simulink model "SDV_HIL"  (R2025a)
settings: Solver=VariableStepAuto  StartTime=0.0  StopTime=9999  FixedStep=0.001  RelTol=1e-3
undefined symbols (not defined in the file): Breakpoints_Fz, Cij, dspblkCoreblockFVToolHelper, eta, Fx_total_max, g, gcbh, Iz, lambda, lf, lr, mu, phi, R_eff, Tmax, xi
libraries: simulink_extras x30, slrealtimeiplib x17, slpidlib x16, simulink x10, SignalEditorBlockLib x6, dspstat3 x5, Solver_SF x3, sl3dlib x3
(part 1 of 5)
settings Model: SimulationMode=accelerator  Creator=zoan  LastModifiedBy=zoan

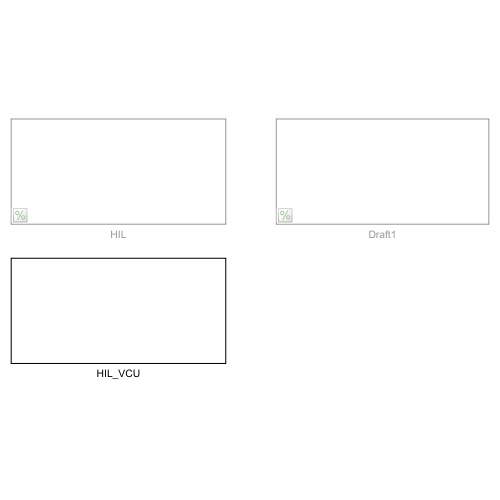
[thumbnail: Simulink's stored preview of the top-level diagram]
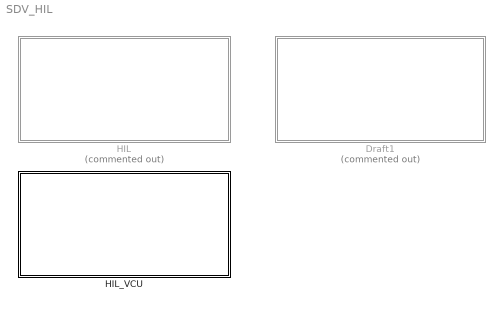
== system SDV_HIL ==
  Draft1 : Subsystem  Commented=on
  HIL : Subsystem  Commented=on
  HIL_VCU : Subsystem

== system SDV_HIL/Draft1 ==
  note: Communication (UDP Protocol)
  CarSim S-Function_video1 : Solver_SF/CarSim S-Function_video  Priority=1  SIMFILE=simfile.sim
      settings: SourceProductName=CarSim S-Function
  Communication System1 : Subsystem  Commented=on
  Connector1 : Subsystem
  Constant3 : Constant  Commented=on  Value=0
  Constant4 : Constant  Commented=on  Value=100
  Custom Trhottle2 : SignalEditorBlockLib/Signal Editor  Commented=on  FileName=Trottle.mat  ActiveScenario=Scenario  ActiveSignal=Signal 1  IsBus=off  OutputBusObjectStr=Bus: BusObject  SampleTime=0  ZeroCross=off  OutputAfterFinalValue=Setting to zero  Unit=inherit  PreserveSignalName=on  ApplySigPropsToAllScenarios=on  ApplySigPropsToAllSignals=off  SignalPropertySource=Dialog parameters
  Data Logger1 : Subsystem
  Driver Logi G1 : Subsystem
  Gain1 : Gain
  Goto2 : Goto  Commented=on  GotoTag=initialCondition  TagVisibility=global
  Sensor1 : Subsystem
  Speed - > Torque1 : Subsystem
  Steering Input1 : Subsystem
  Subsystem1 : Subsystem  Commented=on
  "UDP Receive ZCU -> PC1" : Subsystem
  "UDP Transmit PC -> VCU1" : Subsystem
  VCU Com1 : Subsystem  Commented=on
  tag scope: TqDrive=global
  wires:
  [Fz] -> "UDP Transmit PC -> VCU1"/7(Fz)
  [Vy] -> "UDP Transmit PC -> VCU1"/3(Vy)
  CarSim S-Function_video1/3 -> Sensor1/3(In3)
  [Vx] -> "UDP Transmit PC -> VCU1"/8(Spd)
  Connector1/1(Throttle) -> "UDP Transmit PC -> VCU1"/1(Throttle)
  Speed - > Torque1/1(TqDrive) -> CarSim S-Function_video1/1, [TqDrive]
  "UDP Receive ZCU -> PC1"/1(vxWheel_Ref) -> Speed - > Torque1/1(VxWheel_Ref)
  Steering Input1/1(Str) -> "UDP Transmit PC -> VCU1"/9(Str)
  Gain1/1 -> CarSim S-Function_video1/3
  [ThrottlePXN] -> Connector1/1(In1)
  [Vx] -> "UDP Transmit PC -> VCU1"/2(Vx)
  [yawrate] -> "UDP Transmit PC -> VCU1"/5(r)
  CarSim S-Function_video1/2 -> Sensor1/2(In2)
  Constant3/1 -> Goto2/1
  [Fy] -> "UDP Transmit PC -> VCU1"/6(Fy)
  [Brake_pedal] -> CarSim S-Function_video1/2
  CarSim S-Function_video1/1 -> Sensor1/1(In1)
  [AngWheel] -> "UDP Transmit PC -> VCU1"/4(AngWheel)
  "UDP Receive ZCU -> PC1"/2(AngWheel) -> Gain1/1

== system SDV_HIL/HIL ==
  note: Communication (UDP Protocol)
  CarSim S-Function_video : Solver_SF/CarSim S-Function_video  Priority=1  SIMFILE=simfile.sim
      settings: SourceProductName=CarSim S-Function
  Data Logger : Subsystem
  Driver : Subsystem
  Sensor : Subsystem
  "Speed -> Torque" : Subsystem
  "UDP Receive ZCU -> PC" : Subsystem
  "UDP Transmit PC -> VCU" : Subsystem
  wires:
  [BrakePXN] -> CarSim S-Function_video/2
  CarSim S-Function_video/1 -> Sensor/1(In1)
  "Speed -> Torque"/1(TqDrive) -> CarSim S-Function_video/1
  [Fz] -> "UDP Transmit PC -> VCU"/7(Fz)
  [Fy] -> "UDP Transmit PC -> VCU"/6(Fy)
  [AngWheel] -> "UDP Transmit PC -> VCU"/4(AngWheel)
  [Vx] -> "UDP Transmit PC -> VCU"/8(Spd)
  Driver/1(Throttle) -> "UDP Transmit PC -> VCU"/1(Throttle)
  [Vx] -> "UDP Transmit PC -> VCU"/2(Vx)
  [yawrate] -> "UDP Transmit PC -> VCU"/5(r)
  "UDP Receive ZCU -> PC"/2(AngWheel) -> CarSim S-Function_video/3
  CarSim S-Function_video/2 -> Sensor/2(In2)
  CarSim S-Function_video/3 -> Sensor/3(In3)
  [Vy] -> "UDP Transmit PC -> VCU"/3(Vy)
  "UDP Receive ZCU -> PC"/1(vxWheel_Ref) -> "Speed -> Torque"/1(VxWheel_Ref)
  Driver/2(Steer) -> "UDP Transmit PC -> VCU"/9(Str)

== system SDV_HIL/HIL_VCU ==
  note: Communication (UDP Protocol)
  CarSim S-Function_video : Solver_SF/CarSim S-Function_video  Priority=1  SIMFILE=simfile.sim
      settings: SourceProductName=CarSim S-Function
  Data Logger : Subsystem
  Sensor : Subsystem
  "Speed -> Torque" : Subsystem
  "UDP Receive ZCU -> PC" : Subsystem
  "UDP Receive Brake VCU -> PC" : Subsystem
  "UDP Transmit PC -> VCU" : Subsystem
  wires:
  CarSim S-Function_video/1 -> Sensor/1(In1)
  "Speed -> Torque"/1(TqDrive) -> CarSim S-Function_video/1
  "UDP Receive ZCU -> PC"/2(AngWheel) -> CarSim S-Function_video/3
  CarSim S-Function_video/2 -> Sensor/2(In2)
  CarSim S-Function_video/3 -> Sensor/3(In3)
  "UDP Receive ZCU -> PC"/1(vxWheel_Ref) -> "Speed -> Torque"/1(VxWheel_Ref)
  [Vx] -> "UDP Transmit PC -> VCU"/1(Vx)
  "UDP Receive Brake VCU -> PC"/1(Brake) -> CarSim S-Function_video/2
  [Vy] -> "UDP Transmit PC -> VCU"/2(Vy)
  [AngWheel] -> "UDP Transmit PC -> VCU"/3(AngWheel)
  [yawrate] -> "UDP Transmit PC -> VCU"/4(r)
  [Fz] -> "UDP Transmit PC -> VCU"/5(Fy)
  [Fy] -> "UDP Transmit PC -> VCU"/6(Fz)
  [VxWheel] -> "UDP Transmit PC -> VCU"/7(VxWheel)

== system SDV_HIL/Draft1/Communication System1 ==

== system SDV_HIL/Draft1/Connector1 ==
  In1 : Inport
  Throttle : Outport
  wires:
  In1/1 -> Throttle/1

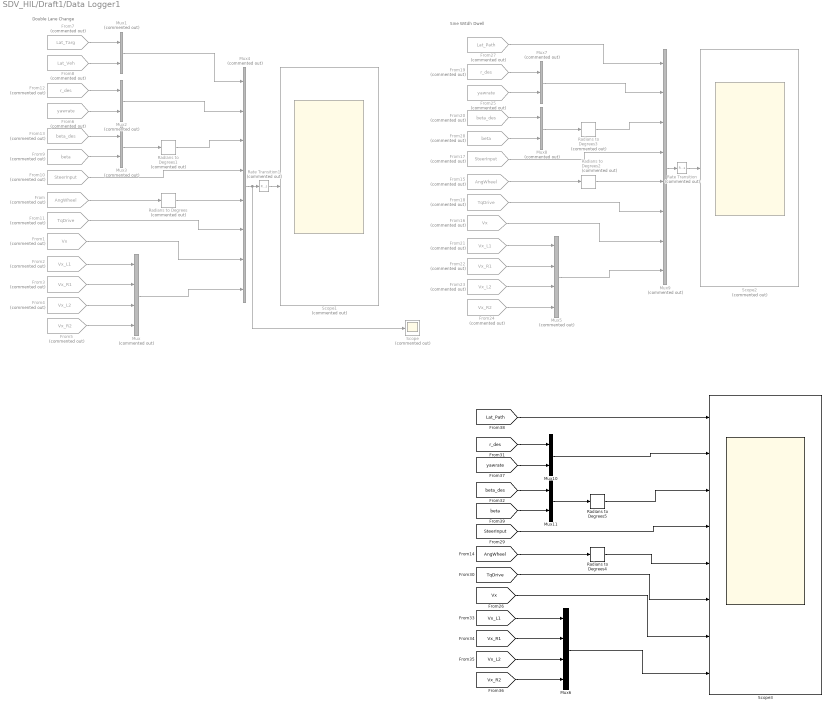
== system SDV_HIL/Draft1/Data Logger1 ==
  note: Sine Witdh Dwell
  note: Double Lane Change
  From : From  Commented=on  GotoTag=AngWheel  TagVisibility=global
  From1 : From  Commented=on  GotoTag=Vx  TagVisibility=global
  From10 : From  Commented=on  GotoTag=SteerInput  TagVisibility=global
  From11 : From  Commented=on  GotoTag=TqDrive  TagVisibility=global
  From12 : From  Commented=on  GotoTag=r_des  TagVisibility=global
  From13 : From  Commented=on  GotoTag=beta_des  TagVisibility=global
  From15 : From  Commented=on  GotoTag=AngWheel  TagVisibility=global
  From16 : From  Commented=on  GotoTag=Vx  TagVisibility=global
  From17 : From  Commented=on  GotoTag=SteerInput  TagVisibility=global
  From18 : From  Commented=on  GotoTag=TqDrive  TagVisibility=global
  From19 : From  Commented=on  GotoTag=r_des  TagVisibility=global
  From2 : From  Commented=on  GotoTag=Vx_L1  TagVisibility=global
  From20 : From  Commented=on  GotoTag=beta_des  TagVisibility=global
  From21 : From  Commented=on  GotoTag=Vx_L1  TagVisibility=global
  From22 : From  Commented=on  GotoTag=Vx_R1  TagVisibility=global
  From23 : From  Commented=on  GotoTag=Vx_L2  TagVisibility=global
  From24 : From  Commented=on  GotoTag=Vx_R2  TagVisibility=global
  From25 : From  Commented=on  GotoTag=yawrate  TagVisibility=global
  From27 : From  Commented=on  GotoTag=Lat_Path  TagVisibility=global
  From28 : From  Commented=on  GotoTag=beta  TagVisibility=global
  From3 : From  Commented=on  GotoTag=Vx_R1  TagVisibility=global
  From4 : From  Commented=on  GotoTag=Vx_L2  TagVisibility=global
  From5 : From  Commented=on  GotoTag=Vx_R2  TagVisibility=global
  From6 : From  Commented=on  GotoTag=yawrate  TagVisibility=global
  From7 : From  Commented=on  GotoTag=Lat_Targ  TagVisibility=global
  From8 : From  Commented=on  GotoTag=Lat_Veh  TagVisibility=global
  From9 : From  Commented=on  GotoTag=beta  TagVisibility=global
  Mux : Mux  Commented=on
  Mux{1..3,7..8} (5 alike) : Mux  Commented=on  Inputs=2
  Mux10 : Mux  Inputs=2
  Mux11 : Mux  Inputs=2
  Mux4 : Mux  Commented=on  Inputs=8
  Mux5 : Mux  Commented=on
  Mux6 : Mux
  Mux9 : Mux  Commented=on  Inputs=8
  Radians to Degrees{,1..3} (4 alike) : simulink_extras/Transformations/Radians to Degrees  Commented=on
  Radians to Degrees4 : simulink_extras/Transformations/Radians to Degrees
  Radians to Degrees5 : simulink_extras/Transformations/Radians to Degrees
  Rate Transition : RateTransition  Commented=on  OutPortSampleTime=0.0005
  Rate Transition1 : RateTransition  Commented=on  OutPortSampleTime=0.0005
  Scope : Scope  Commented=on
      settings: ActiveDisplayYMinimum=-386.40569302982072  ActiveDisplayYMaximum=478.46163200269257  DataLoggingVariableName=ScopeData6
  Scope1 : Scope  Commented=on
      settings: ActiveDisplayYMinimum=-502.14554579924982  ActiveDisplayYMaximum=1193.5717273110276  DataLoggingVariableName=DataPlot
  Scope2 : Scope  Commented=on
      settings: ActiveDisplayYMinimum=90.336925729103882  ActiveDisplayYMaximum=110.69965404556876  DataLoggingVariableName=DataPlot
  Scope3 : Scope  NumInputPorts=8
      settings: ActiveDisplayString=5  ActiveDisplayYMinimum=-20.053815552669828  ActiveDisplayYMaximum=12.34951779667281  YLabel=Wheel Steer angle (deg)  DataLoggingDecimation=10  DataLoggingVariableName=DataPlot1
  wires:
  From/1 -> Radians to Degrees/1
  From2/1 -> Mux/1
  From3/1 -> Mux/2
  From4/1 -> Mux/3
  From5/1 -> Mux/4
  From7/1 -> Mux1/1
  From8/1 -> Mux1/2
  From12/1 -> Mux2/1
  From6/1 -> Mux2/2
  From13/1 -> Mux3/1
  From9/1 -> Mux3/2
  Mux3/1 -> Radians to Degrees1/1
  Mux1/1 -> Mux4/1
  Mux2/1 -> Mux4/2
  Radians to Degrees1/1 -> Mux4/3
  From10/1 -> Mux4/4
  Radians to Degrees/1 -> Mux4/5
  From11/1 -> Mux4/6
  From1/1 -> Mux4/7
  Mux/1 -> Mux4/8
  Mux4/1 -> Scope/1, Rate Transition1/1
  Mux9/1 -> Rate Transition/1
  Mux5/1 -> Mux9/8
  From16/1 -> Mux9/7
  From18/1 -> Mux9/6
  Radians to Degrees2/1 -> Mux9/5
  From17/1 -> Mux9/4
  Radians to Degrees3/1 -> Mux9/3
  Mux7/1 -> Mux9/2
  From27/1 -> Mux9/1
  Mux8/1 -> Radians to Degrees3/1
  From28/1 -> Mux8/2
  From20/1 -> Mux8/1
  From25/1 -> Mux7/2
  From19/1 -> Mux7/1
  From24/1 -> Mux5/4
  From23/1 -> Mux5/3
  From22/1 -> Mux5/2
  From21/1 -> Mux5/1
  From15/1 -> Radians to Degrees2/1
  Rate Transition/1 -> Scope2/1
  Rate Transition1/1 -> Scope1/1
  [AngWheel] -> Radians to Degrees4/1
  [Vx_L1] -> Mux6/1
  [Vx_R1] -> Mux6/2
  [Vx_L2] -> Mux6/3
  [Vx_R2] -> Mux6/4
  [r_des] -> Mux10/1
  [yawrate] -> Mux10/2
  [beta_des] -> Mux11/1
  [beta] -> Mux11/2
  Mux11/1 -> Radians to Degrees5/1
  Radians to Degrees5/1 -> Scope3/3
  [Lat_Path] -> Scope3/1
  Mux10/1 -> Scope3/2
  [SteerInput] -> Scope3/4
  Radians to Degrees4/1 -> Scope3/5
  [TqDrive] -> Scope3/6
  [Vx] -> Scope3/7
  Mux6/1 -> Scope3/8

== system SDV_HIL/Draft1/Driver Logi G1 ==
  Add : Sum
  Add1 : Sum
  Constant : Constant  Value=50
  Constant1 : Constant  Value=6
  Demux : Demux
  Display : Display  Commented=on
  Display1 : Display  Commented=on
  Display{2,4..6} (4 alike) : Display
  Display3 : Display  Commented=on
  Gain3 : Gain  Gain=-6
  Gain4 : Gain  Gain=-50
  Gain5 : Gain  Gain=40
  MATLAB Function : MATLAB Function  TreatAsAtomicUnit=on
  Selector : Selector  InputPortWidth=25  IndexOptions=Index vector (dialog)  Indices=[1]  OutputSizes=1
  Simulation 3D Joystick : sl3dlib/Simulation 3D/Hardware Interface/Simulation 3D Joystick  joyid=1  adjustports=on  forcefeed=off
  Terminator : Terminator
  Terminator2 : Terminator
  tag scope: Brake_pedal=global, SteerPXN=global, ThrottlePXN=global
  wires:
  Simulation 3D Joystick/3 -> Terminator/1
  MATLAB Function/1(state) -> Display4/1
  Selector/1 -> MATLAB Function/1(btn)
  Gain5/1 -> [SteerPXN], Display2/1
  Add1/1 -> Display6/1, [Brake_pedal]
  Constant1/1 -> Add1/2
  Gain3/1 -> Add1/1
  Demux/3 -> Gain3/1
  Demux/2 -> Display3/1, Gain4/1
  Demux/1 -> Gain5/1
  Demux/4 -> Terminator2/1
  Simulation 3D Joystick/1 -> Demux/1, Display/1
  Gain4/1 -> Add/1
  Constant/1 -> Add/2
  Simulation 3D Joystick/2 -> Selector/1, Display1/1
  Add/1 -> Display5/1, [ThrottlePXN]

== system SDV_HIL/Draft1/Sensor1 ==
  In1 : Inport
  In2 : Inport  Port=2
  In3 : Inport  Port=3
  Display : Display  Commented=on
  Display1 : Display  Commented=on
  Display2 : Display  Commented=on
  Steering System : Subsystem
  Torque Vectoring : Subsystem
  Traction Control : Subsystem
  wires:
  In2/1 -> Steering System/1(In1), Display1/1
  In3/1 -> Traction Control/1(In1), Display2/1
  In1/1 -> Torque Vectoring/1(In1), Display/1

== system SDV_HIL/Draft1/Speed - > Torque1 ==
  VxWheel_Ref : Inport
  Demux : Demux
  Gain : Gain  Gain=4
  Mux : Mux
  PID Controller : slpidlib/PID Controller  Controller=PID  Form=Parallel  TimeDomain=Continuous-time  UseExternalTs=off  SampleTime=-1  IntegratorMethod=Forward Euler  FilterMethod=Forward Euler  ControllerParametersSource=internal  P=20  I=0.05  UseKiTs=off  D=1  UseExternalDerivativeSource=off  N=100  UseFilter=on  TunerSelectOption=Transfer Function Based (PID Tuner App)  InitialConditionSource=internal  InitialConditionForIntegrator=0  InitialConditionForFilter=0  DifferentiatorICPrevScaledInput=0  ExternalReset=none  TrackingMode=off  Kt=1  LimitOutput=off  SatLimitsSource=internal  UpperSaturationLimit=inf  LowerSaturationLimit=-inf  LinearizeAsGain=on  AntiWindupMode=none  Kb=1  LimitIntegrator=off  UpperIntegratorSaturationLimit=inf  LowerIntegratorSaturationLimit=-inf  POutMin=[]  POutMax=[]  IOutMin=[]  IOutMax=[]  DOutMin=[]  DOutMax=[]  NOutMin=[]  NOutMax=[]  SumOutMin=[]  SumOutMax=[]  SaturationOutMin=[]  SaturationOutMax=[]  PParamMin=[]  PParamMax=[]  IParamMin=[]  IParamMax=[]  DParamMin=[]  DParamMax=[]  NParamMin=[]  NParamMax=[]  KbParamMin=[]  KbParamMax=[]  KtParamMin=[]  KtParamMax=[]  KbOutMin=[]  KbOutMax=[]  KtOutMin=[]  KtOutMax=[]  IntegratorOutMin=[]  IntegratorOutMax=[]  FilterOutMin=[]  FilterOutMax=[]  SumI1OutMin=[]  SumI1OutMax=[]  SumI2OutMin=[]  SumI2OutMax=[]  SumI3OutMin=[]  SumI3OutMax=[]  SumI4OutMin=[]  SumI4OutMax=[]  SumDOutMin=[]  SumDOutMax=[]  DifferentiatorOutMin=[]  DifferentiatorOutMax=[]  FilterDiffOutCoefMin=[]  FilterDiffOutCoefMax=[]  ReciprocalOutMin=[]  ReciprocalOutMax=[]  SumDenOutMin=[]  SumDenOutMax=[]  SumNumOutMin=[]  SumNumOutMax=[]  DivideOutMin=[]  DivideOutMax=[]  UdiffTsProdOutMin=[]  UdiffTsProdOutMax=[]  NTsProdOutMin=[]  NTsProdOutMax=[]  UintegralTsProdOutMin=[]  UintegralTsProdOutMax=[]  UngainTsProdOutMin=[]  UngainTsProdOutMax=[]  ClampingZeroOutDataTypeStr=Inherit: Inherit via back propagation  ClampingZeroOutMin=[]  ClampingZeroOutMax=[]  FilterDenConstantOutDataTypeStr=Inherit: Inherit via back propagation  FilterDenConstantOutMin=[]  FilterDenConstantOutMax=[]  PCopyOutDataTypeStr=Inherit: Inherit via back propagation  PCopyOutMin=[]  PCopyOutMax=[]  NCopyOutDataTypeStr=Inherit: Inherit via back propagation  NCopyOutMin=[]  NCopyOutMax=[]  IntegratorContinuousStateAttributes=''  IntegratorStateMustResolveToSignalObject=off  IntegratorRTWStateStorageClass=Auto  FilterContinuousStateAttributes=''  FilterStateMustResolveToSignalObject=off  FilterRTWStateStorageClass=Auto  ParallelPVariant=InternalParameters  IdealPVariant=Disabled  IVariant=InternalParameters  DVariant=InternalParameters  IntegratorVariant=Continuous  SatVariant=Disabled  AWVariant=Passthrough  PCopyVariant=Disabled  TRVariant=Disabled  FdbkBlocksVariant=Forward  IdealPFdbkVariant=Disabled  SatFdbkVariant=Disabled  DerivativeFilterVariant=ContFilter  NVariant=InternalParameters  NCopyVariant=Disabled  FilterICVariant=InternalICsFilter  IntegratorICVariant=InternalICs  ExternalResetVariant=Disabled  TRSumVariant=Passthrough  SumFdbkVariant=Disabled  SumVariant=Sum_PID  TsampFilterVariant=InternalTs  TsampNgainVariant=Passthrough  TsampIntegralVariant=Disabled_SignalSpec  ExternalSaturationOutDataTypeStr=Inherit: Same as second input  DerivativeSourceVariant=ErrorSignal  PreIntVariant=InternalPreInt
  Saturation : Saturate  UpperLimit=256  LowerLimit=-256
  Scope : Scope  Commented=on  NumInputPorts=2
      settings: ActiveDisplayYMinimum=-100.56314203320845  ActiveDisplayYMaximum=848.44383025663615  DataLoggingVariableName=ScopeData8
  Scope1 : Scope  Commented=on  NumInputPorts=2
      settings: TimeSpan=10  ActiveDisplayYMinimum=-320  ActiveDisplayYMaximum=320  DataLoggingVariableName=ScopeData15
  Scope2 : Scope  Commented=on
      settings: ActiveDisplayYMinimum=-23.964257405589464  ActiveDisplayYMaximum=18.546534084894063  DataLoggingVariableName=ScopeData34
  Scope4 : Scope  Commented=on
      settings: ActiveDisplayYMinimum=-146.25  ActiveDisplayYMaximum=116.25  DataLoggingVariableName=ScopeData66
  Sum{,1..3} (4 alike) : Sum  Inputs=|+-
  TqDrive : Outport
  wires:
  [Vx_L1] -> Scope/2, Sum/2
  [Vx_R1] -> Sum1/2
  Sum1/1 -> Mux/2
  Sum2/1 -> Mux/3
  [Vx_L2] -> Sum2/2
  Sum3/1 -> Mux/4
  [Vx_R2] -> Sum3/2
  Sum/1 -> Mux/1
  Mux/1 -> Scope2/1, PID Controller/1
  PID Controller/1 -> Saturation/1
  Gain/1 -> Scope1/2, TqDrive/1
  Demux/2 -> Sum1/1
  Demux/3 -> Sum2/1
  Demux/4 -> Sum3/1
  Demux/1 -> Sum/1
  VxWheel_Ref/1 -> Scope4/1, Demux/1
  Saturation/1 -> Scope1/1, Gain/1

== system SDV_HIL/Draft1/Steering Input1 ==
  note: Skenario
  "DLC Lateral Target " : Subsystem  Commented=on
  DLC SteerDM : Subsystem  Commented=on
  Driver Logi G29 : Subsystem  Commented=on
  Gain : Gain  Gain=-1
  Manual Steering : Constant  Commented=on  Value=0
  Scope : Scope  Commented=on
      settings: ActiveDisplayYMinimum=-4.9999999999999991  ActiveDisplayYMaximum=45  DataLoggingVariableName=ScopeData2
  Signal Editor : SignalEditorBlockLib/Signal Editor  Commented=on  FileName=steerDM_DLC_vx100.mat  ActiveScenario=scenario  ActiveSignal=Steering  IsBus=off  OutputBusObjectStr=Bus: BusObject  SampleTime=0  ZeroCross=off  OutputAfterFinalValue=Setting to zero  Unit=inherit  PreserveSignalName=on  ApplySigPropsToAllScenarios=on  ApplySigPropsToAllSignals=off  SignalPropertySource=Dialog parameters
  Sine with Dwell : Subsystem  Commented=on
  Sine with Dwell shifted : Subsystem  Commented=on
  Slider : SliderBlock  ScaleMin=-40  ScaleMax=40
  Steering Custom : SignalEditorBlockLib/Signal Editor  Commented=on  FileName=SteeringTest.mat  ActiveScenario=Scenario  ActiveSignal=Signal 1  IsBus=off  OutputBusObjectStr=Bus: BusObject  SampleTime=0  ZeroCross=off  OutputAfterFinalValue=Setting to zero  Unit=inherit  PreserveSignalName=on  ApplySigPropsToAllScenarios=on  ApplySigPropsToAllSignals=off  SignalPropertySource=Dialog parameters
  Subsystem : Subsystem
  Str : Outport
  tag scope: SteerInput=global
  wires:
  Subsystem/1(Str) -> Str/1, Scope/1, [SteerInput]
  [SteerPXN] -> Gain/1
  Gain/1 -> Subsystem/1(In1)

== system SDV_HIL/Draft1/Subsystem1 ==
  note: Zone Control Unit
  Spd : Inport
  TqWheel : Inport  Port=2
  Mzd : Inport  Port=3
  Ang_reff : Inport  Port=4
  Braking1 : Constant  Value=0
  Motor1 : Subsystem
  Steering1 : Subsystem
      settings: PortSchema="{\"entries\":[{\"content\":{\"sides\":[{\"content\":{\"connectorIds\":[\"In1\"]},\"type\":\"ConnectorPlacement.EquallySpacedRectSide\",\"uuid\":\"adb0bf30-e73b-41b4-a208-76a28c974ff7\"},{\"content\":{\"connectorIds\":[\"Out1\"],\"side\":\"RIGHT\"},\"type\":\"ConnectorPlacement.EquallySpacedRectSide\",\"uuid\":\"cc4abc60-21d6-40e8-bf54-579eb1c50fc1\"},{\"content\":{\"connectorIds\":[\"In2\"],\"side\":\"TOP\"},\"type\":\"ConnectorPlacement.EquallySpacedRectSide\",\"uuid\":\"04732dee-d47d-454e-a8de-965e49d270ff\"}]},\"type\":\"ConnectorPlacement.EquallySpacedConnector\",\"uuid\":\"781362bb-60f7-4755-ab91-304bdf8ac197\"}],\"packageUris\":[\"http://schema.mathworks.com/mf0/Connector/R2020b\"],\"version\":\"1.0\"}"
  Torque to Speed Distribution1 : Subsystem
      settings: PortSchema="{\"entries\":[{\"content\":{\"sides\":[{\"content\":{\"connectorIds\":[\"In1\"]},\"type\":\"ConnectorPlacement.EquallySpacedRectSide\",\"uuid\":\"be15fe61-aaa9-4a20-91d9-47c89f8c78bb\"},{\"content\":{\"connectorIds\":[\"Out1\"],\"side\":\"RIGHT\"},\"type\":\"ConnectorPlacement.EquallySpacedRectSide\",\"uuid\":\"0d489c28-6df0-4c63-af6a-395fd75f26f4\"},{\"content\":{\"connectorIds\":[\"In2\"],\"side\":\"TOP\"},\"type\":\"ConnectorPlacement.EquallySpacedRectSide\",\"uuid\":\"15d17bd3-6c4e-4c2e-8205-0819f815bc2d\"}]},\"type\":\"ConnectorPlacement.EquallySpacedConnector\",\"uuid\":\"9692d941-d4e1-4d2b-a410-04ec1d2de3d9\"}],\"packageUris\":[\"http://schema.mathworks.com/mf0/Connector/R2020b\"],\"version\":\"1.0\"}"
  Out1 : Outport
  Out2 : Outport  Port=2
  Deg : Outport  Port=3
  tag scope: TqDrive=global
  wires:
  Spd/1 -> Torque to Speed Distribution1/2(Spd)
  Motor1/1(Out1) -> Out1/1, [TqDrive]
  Ang_reff/1 -> Steering1/1(Ang_reff)
  Torque to Speed Distribution1/1(SpdWheel) -> Motor1/1(SpdTCS)
  TqWheel/1 -> Torque to Speed Distribution1/1(TqWheel)
  Braking1/1 -> Out2/1
  Mzd/1 -> Steering1/2(Mzd)
  Steering1/1(Deg) -> Deg/1

== system SDV_HIL/Draft1/UDP Receive ZCU -> PC1 ==
  Display18 : Display
  Display26 : Display  Commented=on
  MATLAB Function : MATLAB Function  TreatAsAtomicUnit=on
  Median Filter : dspstat3/Median Filter  Commented=on  WindowLength=5  SimulateUsing=Interpreted execution
      settings: LibrarySourceBlock=|
      | dspfdesign/Median
      | Filter
  Mux : Mux
  Mux1 : Mux
  Rate Transition2 : RateTransition  OutPortSampleTime=0.0001
  Scope : Scope  Commented=on  NumInputPorts=2
      settings: TimeSpan=10  ActiveDisplayYMinimum=-148.76999999999998  ActiveDisplayYMaximum=138.92999999999998  DataLoggingVariableName=ScopeData62
  Scope1 : Scope  Commented=on
      settings: ActiveDisplayYMinimum=-50  ActiveDisplayYMaximum=-30  DataLoggingVariableName=ScopeData63
  Spd & Ang Convertion2 : Subsystem
  UDP Receive3 : slrealtimeiplib/UDP Receive  useHostTargetConn=off  ipAddress=10.252.62.212  localPort=4095  rcvWidth=7  rcvFmAny=on  fmAddress='10.252.62.51'  sampleTime=0.0001  enableMessage=off  maxPackets=1
  vxWheel_Ref : Outport
  AngWheel : Outport  Port=2
  wires:
  MATLAB Function/5(seqRecv) -> Display26/1
  UDP Receive3/2 -> Display18/1
  UDP Receive3/1 -> Rate Transition2/1
  Rate Transition2/1 -> MATLAB Function/1(payload)
  MATLAB Function/4(RR) -> Spd & Ang Convertion2/4(RR)
  MATLAB Function/3(RL) -> Spd & Ang Convertion2/3(RL)
  MATLAB Function/2(FR) -> Spd & Ang Convertion2/2(FR)
  MATLAB Function/1(FL) -> Spd & Ang Convertion2/1(FL)
  Spd & Ang Convertion2/1(ang_FL) -> Mux/1
  Spd & Ang Convertion2/2(ang_FR) -> Mux/2
  Spd & Ang Convertion2/3(ang_RL) -> Mux/3
  Spd & Ang Convertion2/4(ang_RR) -> Mux/4
  Mux/1 -> Scope1/1, AngWheel/1
  Mux1/1 -> Median Filter/1, Scope/1, vxWheel_Ref/1
  Spd & Ang Convertion2/5(vxWheel_FL) -> Mux1/1
  Spd & Ang Convertion2/6(vxWheel_FR) -> Mux1/2
  Spd & Ang Convertion2/7(vxWheel_RL) -> Mux1/3
  Spd & Ang Convertion2/8(vxWheel_RR) -> Mux1/4
  Median Filter/1 -> Scope/2

== system SDV_HIL/Draft1/UDP Transmit PC -> VCU1 ==
  note: UDP Send
      | Matlab -> ZCU
  Throttle : Inport
  Vx : Inport  Port=2
  Vy : Inport  Port=3
  AngWheel : Inport  Port=4
  r : Inport  Port=5
  Fy : Inport  Port=6
  Fz : Inport  Port=7
  Spd : Inport  Port=8
  Str : Inport  Port=9
  Data Type Conversion{,1..3} (4 alike) : DataTypeConversion  OutDataTypeStr=double  SaturateOnIntegerOverflow=off  RndMeth=Floor
  Display{,1,3,5} (4 alike) : Display
  Display4 : Display  Commented=on
  Rate Transition{1..4} (4 alike) : RateTransition  OutPortSampleTime=0.001
  Subsystem : Subsystem
  UDP Send1 : slrealtimeiplib/UDP Send  useHostTargetConn=off  toAddress='10.252.62.51'  toPort=5051  sampleTime=0.001  enableMessage=off  ipAddress=10.252.62.212  localPort=4095
  UDP Send2 : slrealtimeiplib/UDP Send  useHostTargetConn=off  toAddress='10.252.62.52'  toPort=5052  sampleTime=0.001  enableMessage=off  ipAddress=10.252.62.212  localPort=4095
  UDP Send3 : slrealtimeiplib/UDP Send  useHostTargetConn=off  toAddress='10.252.62.53'  toPort=5053  sampleTime=0.001  enableMessage=off  ipAddress=10.252.62.212  localPort=4095
  UDP Send4 : slrealtimeiplib/UDP Send  useHostTargetConn=off  toAddress='10.252.62.54'  toPort=5054  sampleTime=0.001  enableMessage=off  ipAddress=10.252.62.212  localPort=4095
  wires:
  Data Type Conversion2/1 -> UDP Send3/2, Display3/1
  Rate Transition3/1 -> UDP Send3/1
  Rate Transition4/1 -> UDP Send4/1
  Data Type Conversion3/1 -> UDP Send4/2, Display5/1
  Data Type Conversion1/1 -> Display1/1, UDP Send2/2
  Rate Transition2/1 -> UDP Send2/1
  Rate Transition1/1 -> UDP Send1/1
  Data Type Conversion/1 -> UDP Send1/2, Display/1
  Subsystem/1(payload1) -> Display4/1, Rate Transition1/1
  Throttle/1 -> Subsystem/1(Vx_des)
  Vx/1 -> Subsystem/2(Vx)
  Vy/1 -> Subsystem/3(Vy)
  AngWheel/1 -> Subsystem/4(AngWheel)
  r/1 -> Subsystem/5(r)
  Fy/1 -> Subsystem/6(Fy)
  Fz/1 -> Subsystem/7(Fz)
  Spd/1 -> Subsystem/8(Spd)
  Str/1 -> Subsystem/9(Str)
  Subsystem/2(len1) -> Data Type Conversion/1
  Subsystem/3(payload2) -> Rate Transition2/1
  Subsystem/4(len2) -> Data Type Conversion1/1
  Subsystem/5(payload3) -> Rate Transition3/1
  Subsystem/6(len3) -> Data Type Conversion2/1
  Subsystem/7(payload4) -> Rate Transition4/1
  Subsystem/8(len4) -> Data Type Conversion3/1

== system SDV_HIL/Draft1/VCU Com1 ==
  UDP Receive <- VCU1 : Subsystem
  "UDP Send -> VCU1" : Subsystem

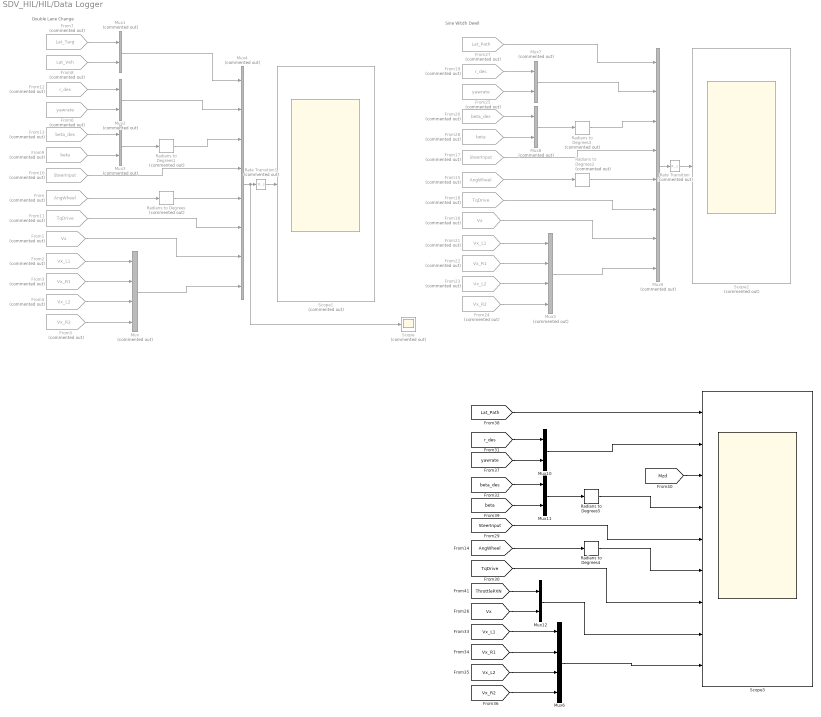
== system SDV_HIL/HIL/Data Logger ==
  note: Sine Witdh Dwell
  note: Double Lane Change
  From : From  Commented=on  GotoTag=AngWheel  TagVisibility=global
  From1 : From  Commented=on  GotoTag=Vx  TagVisibility=global
  From10 : From  Commented=on  GotoTag=SteerInput  TagVisibility=global
  From11 : From  Commented=on  GotoTag=TqDrive  TagVisibility=global
  From12 : From  Commented=on  GotoTag=r_des  TagVisibility=global
  From13 : From  Commented=on  GotoTag=beta_des  TagVisibility=global
  From15 : From  Commented=on  GotoTag=AngWheel  TagVisibility=global
  From16 : From  Commented=on  GotoTag=Vx  TagVisibility=global
  From17 : From  Commented=on  GotoTag=SteerInput  TagVisibility=global
  From18 : From  Commented=on  GotoTag=TqDrive  TagVisibility=global
  From19 : From  Commented=on  GotoTag=r_des  TagVisibility=global
  From2 : From  Commented=on  GotoTag=Vx_L1  TagVisibility=global
  From20 : From  Commented=on  GotoTag=beta_des  TagVisibility=global
  From21 : From  Commented=on  GotoTag=Vx_L1  TagVisibility=global
  From22 : From  Commented=on  GotoTag=Vx_R1  TagVisibility=global
  From23 : From  Commented=on  GotoTag=Vx_L2  TagVisibility=global
  From24 : From  Commented=on  GotoTag=Vx_R2  TagVisibility=global
  From25 : From  Commented=on  GotoTag=yawrate  TagVisibility=global
  From27 : From  Commented=on  GotoTag=Lat_Path  TagVisibility=global
  From28 : From  Commented=on  GotoTag=beta  TagVisibility=global
  From3 : From  Commented=on  GotoTag=Vx_R1  TagVisibility=global
  From4 : From  Commented=on  GotoTag=Vx_L2  TagVisibility=global
  From5 : From  Commented=on  GotoTag=Vx_R2  TagVisibility=global
  From6 : From  Commented=on  GotoTag=yawrate  TagVisibility=global
  From7 : From  Commented=on  GotoTag=Lat_Targ  TagVisibility=global
  From8 : From  Commented=on  GotoTag=Lat_Veh  TagVisibility=global
  From9 : From  Commented=on  GotoTag=beta  TagVisibility=global
  Mux : Mux  Commented=on
  Mux{1..3,7..8} (5 alike) : Mux  Commented=on  Inputs=2
  Mux10 : Mux  Inputs=2
  Mux11 : Mux  Inputs=2
  Mux12 : Mux  Inputs=2
  Mux4 : Mux  Commented=on  Inputs=8
  Mux5 : Mux  Commented=on
  Mux6 : Mux
  Mux9 : Mux  Commented=on  Inputs=8
  Radians to Degrees{,1..3} (4 alike) : simulink_extras/Transformations/Radians to Degrees  Commented=on
  Radians to Degrees4 : simulink_extras/Transformations/Radians to Degrees
  Radians to Degrees5 : simulink_extras/Transformations/Radians to Degrees
  Rate Transition : RateTransition  Commented=on  OutPortSampleTime=0.0005
  Rate Transition1 : RateTransition  Commented=on  OutPortSampleTime=0.0005
  Scope : Scope  Commented=on
      settings: ActiveDisplayYMinimum=-386.40569302982072  ActiveDisplayYMaximum=478.46163200269257  DataLoggingVariableName=ScopeData6
  Scope1 : Scope  Commented=on
      settings: ActiveDisplayYMinimum=-502.14554579924982  ActiveDisplayYMaximum=1193.5717273110276  DataLoggingVariableName=DataPlot
  Scope2 : Scope  Commented=on
      settings: ActiveDisplayYMinimum=90.336925729103882  ActiveDisplayYMaximum=110.69965404556876  DataLoggingVariableName=DataPlot
  Scope3 : Scope  NumInputPorts=9
      settings: TimeSpan=10  ActiveDisplayString=3  ActiveDisplayYMinimum=-593509.73040498013  ActiveDisplayYMaximum=954008.31003345363  YLabel=Mzd (Nm)  DataLoggingDecimation=10  DataLoggingVariableName=DataPlot1
  wires:
  From/1 -> Radians to Degrees/1
  From2/1 -> Mux/1
  From3/1 -> Mux/2
  From4/1 -> Mux/3
  From5/1 -> Mux/4
  From7/1 -> Mux1/1
  From8/1 -> Mux1/2
  From12/1 -> Mux2/1
  From6/1 -> Mux2/2
  From13/1 -> Mux3/1
  From9/1 -> Mux3/2
  Mux3/1 -> Radians to Degrees1/1
  Mux1/1 -> Mux4/1
  Mux2/1 -> Mux4/2
  Radians to Degrees1/1 -> Mux4/3
  From10/1 -> Mux4/4
  Radians to Degrees/1 -> Mux4/5
  From11/1 -> Mux4/6
  From1/1 -> Mux4/7
  Mux/1 -> Mux4/8
  Mux4/1 -> Scope/1, Rate Transition1/1
  Mux9/1 -> Rate Transition/1
  Mux5/1 -> Mux9/8
  From16/1 -> Mux9/7
  From18/1 -> Mux9/6
  Radians to Degrees2/1 -> Mux9/5
  From17/1 -> Mux9/4
  Radians to Degrees3/1 -> Mux9/3
  Mux7/1 -> Mux9/2
  From27/1 -> Mux9/1
  Mux8/1 -> Radians to Degrees3/1
  From28/1 -> Mux8/2
  From20/1 -> Mux8/1
  From25/1 -> Mux7/2
  From19/1 -> Mux7/1
  From24/1 -> Mux5/4
  From23/1 -> Mux5/3
  From22/1 -> Mux5/2
  From21/1 -> Mux5/1
  From15/1 -> Radians to Degrees2/1
  Rate Transition/1 -> Scope2/1
  Rate Transition1/1 -> Scope1/1
  [AngWheel] -> Radians to Degrees4/1
  [Vx_L1] -> Mux6/1
  [Vx_R1] -> Mux6/2
  [Vx_L2] -> Mux6/3
  [Vx_R2] -> Mux6/4
  [r_des] -> Mux10/1
  [yawrate] -> Mux10/2
  [beta_des] -> Mux11/1
  [beta] -> Mux11/2
  Mux11/1 -> Radians to Degrees5/1
  [Lat_Path] -> Scope3/1
  Mux10/1 -> Scope3/2
  Radians to Degrees5/1 -> Scope3/4
  [SteerInput] -> Scope3/5
  Radians to Degrees4/1 -> Scope3/6
  [TqDrive] -> Scope3/7
  Mux6/1 -> Scope3/9
  [Mzd] -> Scope3/3
  [ThrottlePXN] -> Mux12/1
  [Vx] -> Mux12/2
  Mux12/1 -> Scope3/8

== system SDV_HIL/HIL/Driver ==
  note: Skenario
  DLC SteerDM : Subsystem  Commented=on
  Gain : Gain  Gain=-1
  Logitech G29 : Subsystem
  Scope : Scope  Commented=on
      settings: ActiveDisplayYMinimum=-4.9999999999999991  ActiveDisplayYMaximum=45  DataLoggingVariableName=ScopeData2
  Sine with Dwell : Subsystem  Commented=on
  Subsystem : Subsystem
  Throttle : Outport
  Steer : Outport  Port=2
  tag scope: SteerInput=global
  wires:
  Gain/1 -> Subsystem/1(In1)
  [ThrottlePXN] -> Throttle/1
  Subsystem/1(Str) -> [SteerInput], Scope/1, Steer/1
  [SteerPXN] -> Gain/1

== system SDV_HIL/HIL/Sensor ==
  In1 : Inport
  In2 : Inport  Port=2
  In3 : Inport  Port=3
  Display : Display  Commented=on
  Display1 : Display  Commented=on
  Display2 : Display  Commented=on
  Steering System : Subsystem
  Torque Vectoring : Subsystem
  Traction Control : Subsystem
  wires:
  In2/1 -> Steering System/1(In1), Display1/1
  In3/1 -> Traction Control/1(In1), Display2/1
  In1/1 -> Torque Vectoring/1(In1), Display/1

== system SDV_HIL/HIL/Speed -> Torque ==
  VxWheel_Ref : Inport
  Demux : Demux
  Gain : Gain  Gain=4
  Mux : Mux
  PID Controller : slpidlib/PID Controller  Controller=PID  Form=Parallel  TimeDomain=Continuous-time  UseExternalTs=off  SampleTime=-1  IntegratorMethod=Forward Euler  FilterMethod=Forward Euler  ControllerParametersSource=internal  P=20  I=0.05  UseKiTs=off  D=1  UseExternalDerivativeSource=off  N=100  UseFilter=on  TunerSelectOption=Transfer Function Based (PID Tuner App)  InitialConditionSource=internal  InitialConditionForIntegrator=0  InitialConditionForFilter=0  DifferentiatorICPrevScaledInput=0  ExternalReset=none  TrackingMode=off  Kt=1  LimitOutput=off  SatLimitsSource=internal  UpperSaturationLimit=inf  LowerSaturationLimit=-inf  LinearizeAsGain=on  AntiWindupMode=none  Kb=1  LimitIntegrator=off  UpperIntegratorSaturationLimit=inf  LowerIntegratorSaturationLimit=-inf  POutMin=[]  POutMax=[]  IOutMin=[]  IOutMax=[]  DOutMin=[]  DOutMax=[]  NOutMin=[]  NOutMax=[]  SumOutMin=[]  SumOutMax=[]  SaturationOutMin=[]  SaturationOutMax=[]  PParamMin=[]  PParamMax=[]  IParamMin=[]  IParamMax=[]  DParamMin=[]  DParamMax=[]  NParamMin=[]  NParamMax=[]  KbParamMin=[]  KbParamMax=[]  KtParamMin=[]  KtParamMax=[]  KbOutMin=[]  KbOutMax=[]  KtOutMin=[]  KtOutMax=[]  IntegratorOutMin=[]  IntegratorOutMax=[]  FilterOutMin=[]  FilterOutMax=[]  SumI1OutMin=[]  SumI1OutMax=[]  SumI2OutMin=[]  SumI2OutMax=[]  SumI3OutMin=[]  SumI3OutMax=[]  SumI4OutMin=[]  SumI4OutMax=[]  SumDOutMin=[]  SumDOutMax=[]  DifferentiatorOutMin=[]  DifferentiatorOutMax=[]  FilterDiffOutCoefMin=[]  FilterDiffOutCoefMax=[]  ReciprocalOutMin=[]  ReciprocalOutMax=[]  SumDenOutMin=[]  SumDenOutMax=[]  SumNumOutMin=[]  SumNumOutMax=[]  DivideOutMin=[]  DivideOutMax=[]  UdiffTsProdOutMin=[]  UdiffTsProdOutMax=[]  NTsProdOutMin=[]  NTsProdOutMax=[]  UintegralTsProdOutMin=[]  UintegralTsProdOutMax=[]  UngainTsProdOutMin=[]  UngainTsProdOutMax=[]  ClampingZeroOutDataTypeStr=Inherit: Inherit via back propagation  ClampingZeroOutMin=[]  ClampingZeroOutMax=[]  FilterDenConstantOutDataTypeStr=Inherit: Inherit via back propagation  FilterDenConstantOutMin=[]  FilterDenConstantOutMax=[]  PCopyOutDataTypeStr=Inherit: Inherit via back propagation  PCopyOutMin=[]  PCopyOutMax=[]  NCopyOutDataTypeStr=Inherit: Inherit via back propagation  NCopyOutMin=[]  NCopyOutMax=[]  IntegratorContinuousStateAttributes=''  IntegratorStateMustResolveToSignalObject=off  IntegratorRTWStateStorageClass=Auto  FilterContinuousStateAttributes=''  FilterStateMustResolveToSignalObject=off  FilterRTWStateStorageClass=Auto  ParallelPVariant=InternalParameters  IdealPVariant=Disabled  IVariant=InternalParameters  DVariant=InternalParameters  IntegratorVariant=Continuous  SatVariant=Disabled  AWVariant=Passthrough  PCopyVariant=Disabled  TRVariant=Disabled  FdbkBlocksVariant=Forward  IdealPFdbkVariant=Disabled  SatFdbkVariant=Disabled  DerivativeFilterVariant=ContFilter  NVariant=InternalParameters  NCopyVariant=Disabled  FilterICVariant=InternalICsFilter  IntegratorICVariant=InternalICs  ExternalResetVariant=Disabled  TRSumVariant=Passthrough  SumFdbkVariant=Disabled  SumVariant=Sum_PID  TsampFilterVariant=InternalTs  TsampNgainVariant=Passthrough  TsampIntegralVariant=Disabled_SignalSpec  ExternalSaturationOutDataTypeStr=Inherit: Same as second input  DerivativeSourceVariant=ErrorSignal  PreIntVariant=InternalPreInt
  Saturation : Saturate  UpperLimit=256  LowerLimit=-100
  Scope : Scope  Commented=on  NumInputPorts=2
      settings: ActiveDisplayYMinimum=-100.56314203320845  ActiveDisplayYMaximum=848.44383025663615  DataLoggingVariableName=ScopeData8
  Scope1 : Scope  Commented=on  NumInputPorts=2
      settings: TimeSpan=10  ActiveDisplayYMinimum=-320  ActiveDisplayYMaximum=320  DataLoggingVariableName=ScopeData15
  Scope2 : Scope  Commented=on
      settings: ActiveDisplayYMinimum=-23.964257405589464  ActiveDisplayYMaximum=18.546534084894063  DataLoggingVariableName=ScopeData34
  Scope4 : Scope  Commented=on
      settings: ActiveDisplayYMinimum=-146.25  ActiveDisplayYMaximum=116.25  DataLoggingVariableName=ScopeData66
  Sum{,1..3} (4 alike) : Sum  Inputs=|+-
  TqDrive : Outport
  tag scope: TqDrive=global
  wires:
  [Vx_L1] -> Scope/2, Sum/2
  [Vx_R1] -> Sum1/2
  Sum1/1 -> Mux/2
  Sum2/1 -> Mux/3
  [Vx_L2] -> Sum2/2
  Sum3/1 -> Mux/4
  [Vx_R2] -> Sum3/2
  Sum/1 -> Mux/1
  Mux/1 -> Scope2/1, PID Controller/1
  PID Controller/1 -> Saturation/1
  Gain/1 -> [TqDrive], Scope1/2, TqDrive/1
  Demux/2 -> Sum1/1
  Demux/3 -> Sum2/1
  Demux/4 -> Sum3/1
  Demux/1 -> Sum/1
  VxWheel_Ref/1 -> Scope4/1, Demux/1
  Saturation/1 -> Scope1/1, Gain/1

== system SDV_HIL/HIL/UDP Receive ZCU -> PC ==
  Display18 : Display
  Display26 : Display  Commented=on
  Gain1 : Gain  Gain=-1
  MATLAB Function : MATLAB Function  TreatAsAtomicUnit=on
  Median Filter : dspstat3/Median Filter  Commented=on  WindowLength=5  SimulateUsing=Interpreted execution
      settings: LibrarySourceBlock=|
      | dspfdesign/Median
      | Filter
  Mux : Mux
  Mux1 : Mux
  Rate Transition2 : RateTransition  OutPortSampleTime=0.0001
  Scope : Scope  Commented=on  NumInputPorts=2
      settings: TimeSpan=10  ActiveDisplayYMinimum=-148.76999999999998  ActiveDisplayYMaximum=138.92999999999998  DataLoggingVariableName=ScopeData62
  Scope1 : Scope  Commented=on
      settings: ActiveDisplayYMinimum=-50  ActiveDisplayYMaximum=-30  DataLoggingVariableName=ScopeData63
  Spd & Ang Convertion2 : Subsystem
  UDP Receive3 : slrealtimeiplib/UDP Receive  useHostTargetConn=off  ipAddress=10.252.62.212  localPort=4095  rcvWidth=7  rcvFmAny=on  fmAddress='10.252.62.51'  sampleTime=0.0001  enableMessage=off  maxPackets=1
  vxWheel_Ref : Outport
  AngWheel : Outport  Port=2
  wires:
  MATLAB Function/5(seqRecv) -> Display26/1
  UDP Receive3/2 -> Display18/1
  UDP Receive3/1 -> Rate Transition2/1
  Rate Transition2/1 -> MATLAB Function/1(payload)
  MATLAB Function/4(RR) -> Spd & Ang Convertion2/4(RR)
  MATLAB Function/3(RL) -> Spd & Ang Convertion2/3(RL)
  MATLAB Function/2(FR) -> Spd & Ang Convertion2/2(FR)
  MATLAB Function/1(FL) -> Spd & Ang Convertion2/1(FL)
  Spd & Ang Convertion2/1(ang_FL) -> Mux/1
  Spd & Ang Convertion2/2(ang_FR) -> Mux/2
  Spd & Ang Convertion2/3(ang_RL) -> Mux/3
  Spd & Ang Convertion2/4(ang_RR) -> Mux/4
  Mux/1 -> Gain1/1
  Spd & Ang Convertion2/5(vxWheel_FL) -> Mux1/1
  Spd & Ang Convertion2/6(vxWheel_FR) -> Mux1/2
  Spd & Ang Convertion2/7(vxWheel_RL) -> Mux1/3
  Spd & Ang Convertion2/8(vxWheel_RR) -> Mux1/4
  Median Filter/1 -> Scope/2
  Mux1/1 -> Median Filter/1, vxWheel_Ref/1, Scope/1
  Gain1/1 -> Scope1/1, AngWheel/1

== system SDV_HIL/HIL/UDP Transmit PC -> VCU ==
  note: UDP Send
      | Matlab -> ZCU
  Throttle : Inport
  Vx : Inport  Port=2
  Vy : Inport  Port=3
  AngWheel : Inport  Port=4
  r : Inport  Port=5
  Fy : Inport  Port=6
  Fz : Inport  Port=7
  Spd : Inport  Port=8
  Str : Inport  Port=9
  Data Type Conversion{,1..3} (4 alike) : DataTypeConversion  OutDataTypeStr=double  SaturateOnIntegerOverflow=off  RndMeth=Floor
  Display{,1,3,5} (4 alike) : Display
  Display4 : Display  Commented=on
  Gain1 : Gain  Gain=-1
  Rate Transition{1..4} (4 alike) : RateTransition  OutPortSampleTime=0.001
  Subsystem : Subsystem
  UDP Send1 : slrealtimeiplib/UDP Send  useHostTargetConn=off  toAddress='10.252.62.51'  toPort=5051  sampleTime=0.001  enableMessage=off  ipAddress=10.252.62.212  localPort=4095
  UDP Send2 : slrealtimeiplib/UDP Send  useHostTargetConn=off  toAddress='10.252.62.52'  toPort=5052  sampleTime=0.001  enableMessage=off  ipAddress=10.252.62.212  localPort=4095
  UDP Send3 : slrealtimeiplib/UDP Send  useHostTargetConn=off  toAddress='10.252.62.53'  toPort=5053  sampleTime=0.001  enableMessage=off  ipAddress=10.252.62.212  localPort=4095
  UDP Send4 : slrealtimeiplib/UDP Send  useHostTargetConn=off  toAddress='10.252.62.54'  toPort=5054  sampleTime=0.001  enableMessage=off  ipAddress=10.252.62.212  localPort=4095
  wires:
  Data Type Conversion2/1 -> UDP Send3/2, Display3/1
  Rate Transition3/1 -> UDP Send3/1
  Rate Transition4/1 -> UDP Send4/1
  Data Type Conversion3/1 -> UDP Send4/2, Display5/1
  Data Type Conversion1/1 -> Display1/1, UDP Send2/2
  Rate Transition2/1 -> UDP Send2/1
  Rate Transition1/1 -> UDP Send1/1
  Data Type Conversion/1 -> UDP Send1/2, Display/1
  Subsystem/1(payload1) -> Display4/1, Rate Transition1/1
  Throttle/1 -> Subsystem/1(Vx_des)
  Vx/1 -> Subsystem/2(Vx)
  Vy/1 -> Subsystem/3(Vy)
  r/1 -> Subsystem/5(r)
  Fy/1 -> Subsystem/6(Fy)
  Fz/1 -> Subsystem/7(Fz)
  Spd/1 -> Subsystem/8(Spd)
  Str/1 -> Gain1/1
  Subsystem/2(len1) -> Data Type Conversion/1
  Subsystem/3(payload2) -> Rate Transition2/1
  Subsystem/4(len2) -> Data Type Conversion1/1
  Subsystem/5(payload3) -> Rate Transition3/1
  Subsystem/6(len3) -> Data Type Conversion2/1
  Subsystem/7(payload4) -> Rate Transition4/1
  Subsystem/8(len4) -> Data Type Conversion3/1
  AngWheel/1 -> Subsystem/4(AngWheel)
  Gain1/1 -> Subsystem/9(Str)

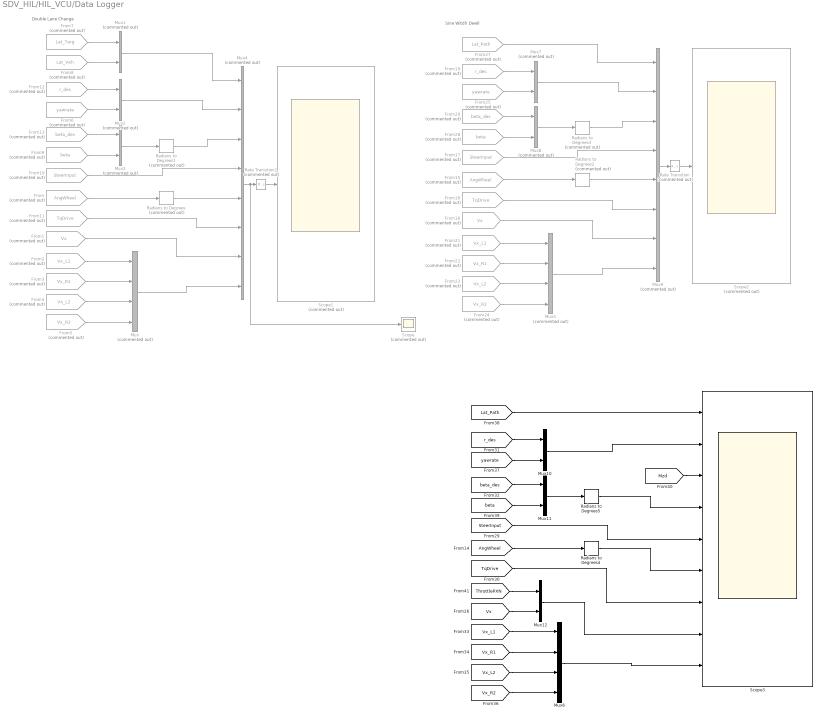
== system SDV_HIL/HIL_VCU/Data Logger ==
  note: Sine Witdh Dwell
  note: Double Lane Change
  From : From  Commented=on  GotoTag=AngWheel  TagVisibility=global
  From1 : From  Commented=on  GotoTag=Vx  TagVisibility=global
  From10 : From  Commented=on  GotoTag=SteerInput  TagVisibility=global
  From11 : From  Commented=on  GotoTag=TqDrive  TagVisibility=global
  From12 : From  Commented=on  GotoTag=r_des  TagVisibility=global
  From13 : From  Commented=on  GotoTag=beta_des  TagVisibility=global
  From15 : From  Commented=on  GotoTag=AngWheel  TagVisibility=global
  From16 : From  Commented=on  GotoTag=Vx  TagVisibility=global
  From17 : From  Commented=on  GotoTag=SteerInput  TagVisibility=global
  From18 : From  Commented=on  GotoTag=TqDrive  TagVisibility=global
  From19 : From  Commented=on  GotoTag=r_des  TagVisibility=global
  From2 : From  Commented=on  GotoTag=Vx_L1  TagVisibility=global
  From20 : From  Commented=on  GotoTag=beta_des  TagVisibility=global
  From21 : From  Commented=on  GotoTag=Vx_L1  TagVisibility=global
  From22 : From  Commented=on  GotoTag=Vx_R1  TagVisibility=global
  From23 : From  Commented=on  GotoTag=Vx_L2  TagVisibility=global
  From24 : From  Commented=on  GotoTag=Vx_R2  TagVisibility=global
  From25 : From  Commented=on  GotoTag=yawrate  TagVisibility=global
  From27 : From  Commented=on  GotoTag=Lat_Path  TagVisibility=global
  From28 : From  Commented=on  GotoTag=beta  TagVisibility=global
  From3 : From  Commented=on  GotoTag=Vx_R1  TagVisibility=global
  From4 : From  Commented=on  GotoTag=Vx_L2  TagVisibility=global
  From5 : From  Commented=on  GotoTag=Vx_R2  TagVisibility=global
  From6 : From  Commented=on  GotoTag=yawrate  TagVisibility=global
  From7 : From  Commented=on  GotoTag=Lat_Targ  TagVisibility=global
  From8 : From  Commented=on  GotoTag=Lat_Veh  TagVisibility=global
  From9 : From  Commented=on  GotoTag=beta  TagVisibility=global
  Mux : Mux  Commented=on
  Mux{1..3,7..8} (5 alike) : Mux  Commented=on  Inputs=2
  Mux10 : Mux  Inputs=2
  Mux11 : Mux  Inputs=2
  Mux12 : Mux  Inputs=2
  Mux4 : Mux  Commented=on  Inputs=8
  Mux5 : Mux  Commented=on
  Mux6 : Mux
  Mux9 : Mux  Commented=on  Inputs=8
  Radians to Degrees{,1..3} (4 alike) : simulink_extras/Transformations/Radians to Degrees  Commented=on
  Radians to Degrees4 : simulink_extras/Transformations/Radians to Degrees
  Radians to Degrees5 : simulink_extras/Transformations/Radians to Degrees
  Rate Transition : RateTransition  Commented=on  OutPortSampleTime=0.0005
  Rate Transition1 : RateTransition  Commented=on  OutPortSampleTime=0.0005
  Scope : Scope  Commented=on
      settings: ActiveDisplayYMinimum=-386.40569302982072  ActiveDisplayYMaximum=478.46163200269257  DataLoggingVariableName=ScopeData6
  Scope1 : Scope  Commented=on
      settings: ActiveDisplayYMinimum=-502.14554579924982  ActiveDisplayYMaximum=1193.5717273110276  DataLoggingVariableName=DataPlot
  Scope2 : Scope  Commented=on
      settings: ActiveDisplayYMinimum=90.336925729103882  ActiveDisplayYMaximum=110.69965404556876  DataLoggingVariableName=DataPlot
  Scope3 : Scope  NumInputPorts=9
      settings: TimeSpan=10  ActiveDisplayYMinimum=-0.086550065129143511  ActiveDisplayYMaximum=0.051008431956528627  YLabel=Yaw rate (rad/s)  DataLoggingDecimation=10  DataLoggingVariableName=DataPlot1
  wires:
  From/1 -> Radians to Degrees/1
  From2/1 -> Mux/1
  From3/1 -> Mux/2
  From4/1 -> Mux/3
  From5/1 -> Mux/4
  From7/1 -> Mux1/1
  From8/1 -> Mux1/2
  From12/1 -> Mux2/1
  From6/1 -> Mux2/2
  From13/1 -> Mux3/1
  From9/1 -> Mux3/2
  Mux3/1 -> Radians to Degrees1/1
  Mux1/1 -> Mux4/1
  Mux2/1 -> Mux4/2
  Radians to Degrees1/1 -> Mux4/3
  From10/1 -> Mux4/4
  Radians to Degrees/1 -> Mux4/5
  From11/1 -> Mux4/6
  From1/1 -> Mux4/7
  Mux/1 -> Mux4/8
  Mux4/1 -> Scope/1, Rate Transition1/1
  Mux9/1 -> Rate Transition/1
  Mux5/1 -> Mux9/8
  From16/1 -> Mux9/7
  From18/1 -> Mux9/6
  Radians to Degrees2/1 -> Mux9/5
  From17/1 -> Mux9/4
  Radians to Degrees3/1 -> Mux9/3
  Mux7/1 -> Mux9/2
  From27/1 -> Mux9/1
  Mux8/1 -> Radians to Degrees3/1
  From28/1 -> Mux8/2
  From20/1 -> Mux8/1
  From25/1 -> Mux7/2
  From19/1 -> Mux7/1
  From24/1 -> Mux5/4
  From23/1 -> Mux5/3
  From22/1 -> Mux5/2
  From21/1 -> Mux5/1
  From15/1 -> Radians to Degrees2/1
  Rate Transition/1 -> Scope2/1
  Rate Transition1/1 -> Scope1/1
  [AngWheel] -> Radians to Degrees4/1
  [Vx_L1] -> Mux6/1
  [Vx_R1] -> Mux6/2
  [Vx_L2] -> Mux6/3
  [Vx_R2] -> Mux6/4
  [r_des] -> Mux10/1
  [yawrate] -> Mux10/2
  [beta_des] -> Mux11/1
  [beta] -> Mux11/2
  Mux11/1 -> Radians to Degrees5/1
  [Lat_Path] -> Scope3/1
  Mux10/1 -> Scope3/2
  Radians to Degrees5/1 -> Scope3/4
  [SteerInput] -> Scope3/5
  Radians to Degrees4/1 -> Scope3/6
  [TqDrive] -> Scope3/7
  Mux6/1 -> Scope3/9
  [Mzd] -> Scope3/3
  [ThrottlePXN] -> Mux12/1
  [Vx] -> Mux12/2
  Mux12/1 -> Scope3/8

== system SDV_HIL/HIL_VCU/Sensor ==
  In1 : Inport
  In2 : Inport  Port=2
  In3 : Inport  Port=3
  Display : Display  Commented=on
  Display1 : Display  Commented=on
  Display2 : Display  Commented=on
  Steering System : Subsystem
  Torque Vectoring : Subsystem
  Traction Control : Subsystem
  wires:
  In2/1 -> Steering System/1(In1), Display1/1
  In3/1 -> Traction Control/1(In1), Display2/1
  In1/1 -> Torque Vectoring/1(In1), Display/1

== system SDV_HIL/HIL_VCU/Speed -> Torque ==
  VxWheel_Ref : Inport
  Demux : Demux
  Gain : Gain  Gain=4
  Mux : Mux
  PID Controller : slpidlib/PID Controller  Controller=PID  Form=Parallel  TimeDomain=Continuous-time  UseExternalTs=off  SampleTime=-1  IntegratorMethod=Forward Euler  FilterMethod=Forward Euler  ControllerParametersSource=internal  P=20  I=0.05  UseKiTs=off  D=1  UseExternalDerivativeSource=off  N=100  UseFilter=on  TunerSelectOption=Transfer Function Based (PID Tuner App)  InitialConditionSource=internal  InitialConditionForIntegrator=0  InitialConditionForFilter=0  DifferentiatorICPrevScaledInput=0  ExternalReset=none  TrackingMode=off  Kt=1  LimitOutput=off  SatLimitsSource=internal  UpperSaturationLimit=inf  LowerSaturationLimit=-inf  LinearizeAsGain=on  AntiWindupMode=none  Kb=1  LimitIntegrator=off  UpperIntegratorSaturationLimit=inf  LowerIntegratorSaturationLimit=-inf  POutMin=[]  POutMax=[]  IOutMin=[]  IOutMax=[]  DOutMin=[]  DOutMax=[]  NOutMin=[]  NOutMax=[]  SumOutMin=[]  SumOutMax=[]  SaturationOutMin=[]  SaturationOutMax=[]  PParamMin=[]  PParamMax=[]  IParamMin=[]  IParamMax=[]  DParamMin=[]  DParamMax=[]  NParamMin=[]  NParamMax=[]  KbParamMin=[]  KbParamMax=[]  KtParamMin=[]  KtParamMax=[]  KbOutMin=[]  KbOutMax=[]  KtOutMin=[]  KtOutMax=[]  IntegratorOutMin=[]  IntegratorOutMax=[]  FilterOutMin=[]  FilterOutMax=[]  SumI1OutMin=[]  SumI1OutMax=[]  SumI2OutMin=[]  SumI2OutMax=[]  SumI3OutMin=[]  SumI3OutMax=[]  SumI4OutMin=[]  SumI4OutMax=[]  SumDOutMin=[]  SumDOutMax=[]  DifferentiatorOutMin=[]  DifferentiatorOutMax=[]  FilterDiffOutCoefMin=[]  FilterDiffOutCoefMax=[]  ReciprocalOutMin=[]  ReciprocalOutMax=[]  SumDenOutMin=[]  SumDenOutMax=[]  SumNumOutMin=[]  SumNumOutMax=[]  DivideOutMin=[]  DivideOutMax=[]  UdiffTsProdOutMin=[]  UdiffTsProdOutMax=[]  NTsProdOutMin=[]  NTsProdOutMax=[]  UintegralTsProdOutMin=[]  UintegralTsProdOutMax=[]  UngainTsProdOutMin=[]  UngainTsProdOutMax=[]  ClampingZeroOutDataTypeStr=Inherit: Inherit via back propagation  ClampingZeroOutMin=[]  ClampingZeroOutMax=[]  FilterDenConstantOutDataTypeStr=Inherit: Inherit via back propagation  FilterDenConstantOutMin=[]  FilterDenConstantOutMax=[]  PCopyOutDataTypeStr=Inherit: Inherit via back propagation  PCopyOutMin=[]  PCopyOutMax=[]  NCopyOutDataTypeStr=Inherit: Inherit via back propagation  NCopyOutMin=[]  NCopyOutMax=[]  IntegratorContinuousStateAttributes=''  IntegratorStateMustResolveToSignalObject=off  IntegratorRTWStateStorageClass=Auto  FilterContinuousStateAttributes=''  FilterStateMustResolveToSignalObject=off  FilterRTWStateStorageClass=Auto  ParallelPVariant=InternalParameters  IdealPVariant=Disabled  IVariant=InternalParameters  DVariant=InternalParameters  IntegratorVariant=Continuous  SatVariant=Disabled  AWVariant=Passthrough  PCopyVariant=Disabled  TRVariant=Disabled  FdbkBlocksVariant=Forward  IdealPFdbkVariant=Disabled  SatFdbkVariant=Disabled  DerivativeFilterVariant=ContFilter  NVariant=InternalParameters  NCopyVariant=Disabled  FilterICVariant=InternalICsFilter  IntegratorICVariant=InternalICs  ExternalResetVariant=Disabled  TRSumVariant=Passthrough  SumFdbkVariant=Disabled  SumVariant=Sum_PID  TsampFilterVariant=InternalTs  TsampNgainVariant=Passthrough  TsampIntegralVariant=Disabled_SignalSpec  ExternalSaturationOutDataTypeStr=Inherit: Same as second input  DerivativeSourceVariant=ErrorSignal  PreIntVariant=InternalPreInt
  Saturation : Saturate  UpperLimit=256  LowerLimit=-100
  Scope : Scope  Commented=on  NumInputPorts=2
      settings: ActiveDisplayYMinimum=-100.56314203320845  ActiveDisplayYMaximum=848.44383025663615  DataLoggingVariableName=ScopeData8
  Scope1 : Scope  Commented=on  NumInputPorts=2
      settings: TimeSpan=10  ActiveDisplayYMinimum=-320  ActiveDisplayYMaximum=320  DataLoggingVariableName=ScopeData15
  Scope2 : Scope  Commented=on
      settings: ActiveDisplayYMinimum=-23.964257405589464  ActiveDisplayYMaximum=18.546534084894063  DataLoggingVariableName=ScopeData34
  Scope4 : Scope  Commented=on
      settings: ActiveDisplayYMinimum=-146.25  ActiveDisplayYMaximum=116.25  DataLoggingVariableName=ScopeData66
  Sum{,1..3} (4 alike) : Sum  Inputs=|+-
  TqDrive : Outport
  tag scope: TqDrive=global
  wires:
  [Vx_L1] -> Scope/2, Sum/2
  [Vx_R1] -> Sum1/2
  Sum1/1 -> Mux/2
  Sum2/1 -> Mux/3
  [Vx_L2] -> Sum2/2
  Sum3/1 -> Mux/4
  [Vx_R2] -> Sum3/2
  Sum/1 -> Mux/1
  Mux/1 -> Scope2/1, PID Controller/1
  PID Controller/1 -> Saturation/1
  Gain/1 -> [TqDrive], Scope1/2, TqDrive/1
  Demux/2 -> Sum1/1
  Demux/3 -> Sum2/1
  Demux/4 -> Sum3/1
  Demux/1 -> Sum/1
  VxWheel_Ref/1 -> Scope4/1, Demux/1
  Saturation/1 -> Scope1/1, Gain/1
